simulink model "ParkPrdct"  (Simulink 7.5)
settings: Solver=ode45  StartTime=0.0  StopTime=10.0  FixedStep=0.01  RelTol=1e-3
settings Model: Creator=Dranik_win  LastModifiedBy=Dranik_win
settings SolverCC: InitialStep=0.001

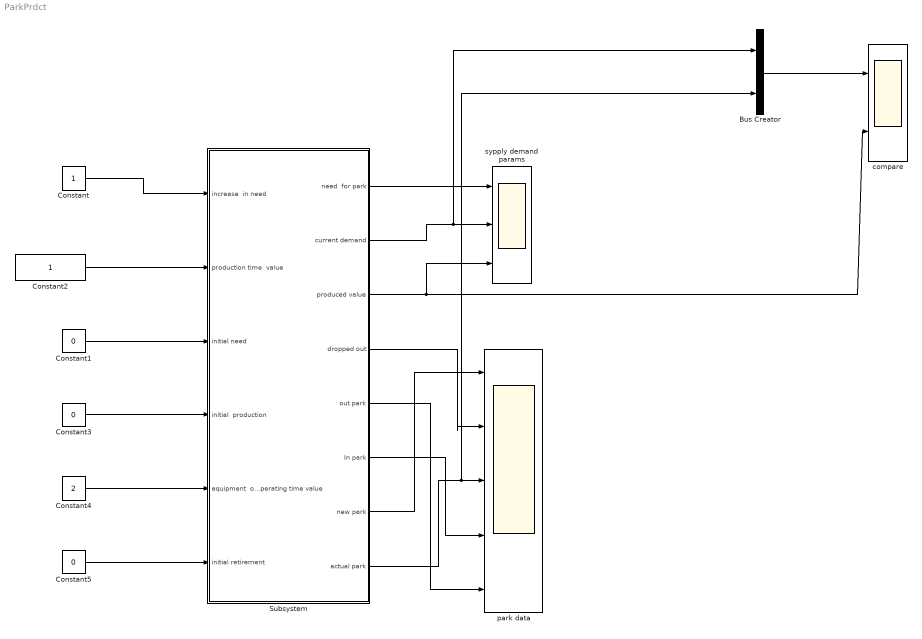
== system ParkPrdct ==
  Bus Creator : BusCreator  Inputs=2
  Constant : Constant  OutDataType=fixdt(1, 16)  OutScaling=2^0
  Constant1 : Constant  Value=0  OutDataType=fixdt(1, 16)  OutScaling=2^0
  Constant2 : Constant  OutDataType=fixdt(1, 16)  OutScaling=2^0
  Constant3 : Constant  Value=0  OutDataType=fixdt(1, 16)  OutScaling=2^0
  Constant4 : Constant  Value=2  VectorParams1D=off  OutDataType=fixdt(1, 16)  OutScaling=2^0
  Constant5 : Constant  Value=0  OutDataType=fixdt(1, 16)  OutScaling=2^0
  Subsystem : Subsystem
  compare : Scope  NumInputPorts=2
      settings: YMin=-5~-5  YMax=5~5  SaveName=ScopeData2
  park data : Scope  NumInputPorts=5
      settings: YMin=-5~-5~-5~-5~-5  YMax=5~5~5~5~5
  sypply demand params : Scope  NumInputPorts=3
      settings: YMin=-5~-5~-5  YMax=5~5~5
  wires:
  Constant/1 -> Subsystem/1(increase  in need)
  Constant1/1 -> Subsystem/3(initial need)
  Constant2/1 -> Subsystem/2(production time  value)
  Constant3/1 -> Subsystem/4(initial  production)
  Constant4/1 -> Subsystem/5(equipment  operating time value)
  Constant5/1 -> Subsystem/6(initial retirement)
  Subsystem/7(new park) -> park data/1
  Subsystem/4(dropped out) -> park data/2
  Subsystem/8(actual park) -> park data/3, Bus Creator/2
  Subsystem/6(In park) -> park data/4
  Subsystem/5(out park) -> park data/5
  Subsystem/1(need  for park) -> sypply demand params/1
  Subsystem/2(current demand) -> sypply demand params/2, Bus Creator/1
  Subsystem/3(produced value) -> sypply demand params/3, compare/2
  Bus Creator/1 -> compare/1

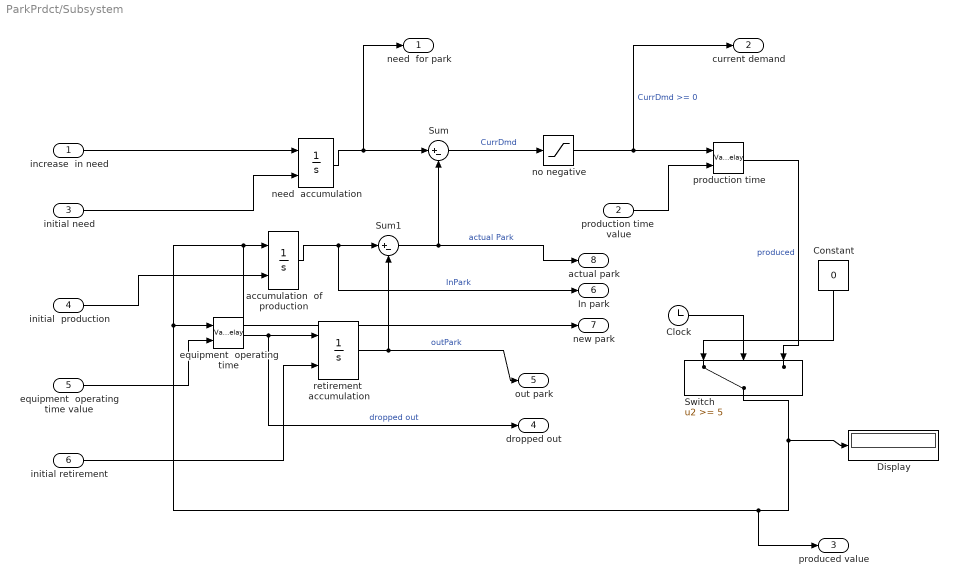
== system ParkPrdct/Subsystem ==
  increase  in need : Inport  OutDataType=fixdt(1, 16)  OutScaling=2^0
  production time  value : Inport  Port=2  OutDataType=fixdt(1, 16)  OutScaling=2^0
  initial need : Inport  Port=3  OutDataType=fixdt(1, 16)  OutScaling=2^0
  initial  production : Inport  Port=4  OutDataType=fixdt(1, 16)  OutScaling=2^0
  equipment  operating time value : Inport  Port=5  OutDataType=fixdt(1, 16)  OutScaling=2^0
  initial retirement : Inport  Port=6  OutDataType=fixdt(1, 16)  OutScaling=2^0
  Clock : Clock
      settings: Decimation=10
  Constant : Constant  Value=0  OutDataType=fixdt(1, 16)  OutScaling=2^0
  Display : Display
  Sum : Sum  Inputs=|+-  OutDataType=fixdt(1, 16)  OutScaling=2^0
  Sum1 : Sum  Inputs=|+-  OutDataType=fixdt(1, 16)  OutScaling=2^0
  Switch : Switch  Threshold=5  OutDataType=fixdt(1, 16)  OutScaling=2^0
  accumulation  of production : Integrator  InitialConditionSource=external
  equipment  operating time : VariableTransportDelay  VariableDelayType=Variable transport delay  MaximumDelay=10
  need  accumulation : Integrator  InitialConditionSource=external
  no negative : Saturate  UpperLimit=Inf  LowerLimit=0  OutDataType=fixdt(1, 16)  OutScaling=2^0
  production time : VariableTransportDelay  VariableDelayType=Variable transport delay  MaximumDelay=10
  retirement  accumulation : Integrator  InitialConditionSource=external
  need  for park : Outport  OutDataType=fixdt(1, 16)  OutScaling=2^0
  current demand : Outport  Port=2  OutDataType=fixdt(1, 16)  OutScaling=2^0
  produced value : Outport  Port=3  OutDataType=fixdt(1, 16)  OutScaling=2^0
  dropped out : Outport  Port=4
  out park : Outport  Port=5
  In park : Outport  Port=6
  new park : Outport  Port=7
  actual park : Outport  Port=8
  wires:
  increase  in need/1 -> need  accumulation/1
  need  accumulation/1 -> need  for park/1, Sum/1
  Sum/1 -> no negative/1  "CurrDmd"
  no negative/1 -> production time/1, current demand/1  "CurrDmd >= 0"
  production time  value/1 -> production time/2
  initial need/1 -> need  accumulation/2
  production time/1 -> Switch/3  "produced"
  equipment  operating time value/1 -> equipment  operating time/2
  Sum1/1 -> Sum/2, actual park/1  "actual Park"
  equipment  operating time/1 -> retirement  accumulation/1, dropped out/1  "dropped out"
  retirement  accumulation/1 -> Sum1/2, out park/1  "outPark"
  initial retirement/1 -> retirement  accumulation/2
  accumulation  of production/1 -> Sum1/1, In park/1  "InPark"
  initial  production/1 -> accumulation  of production/2
  Switch/1 -> Display/1, equipment  operating time/1, accumulation  of production/1, new park/1, produced value/1
  Clock/1 -> Switch/2
  Constant/1 -> Switch/1
